simulink model "Sim_PD_XY"  (R2016a)
settings: Solver=VariableStepAuto  StartTime=0.0  StopTime=10.0  RelTol=1e-3
undefined symbols (not defined in the file or in its folder): k_reg, k_s, T_n, T_r
settings Model: Creator=Florian  LastModifiedBy=Florian

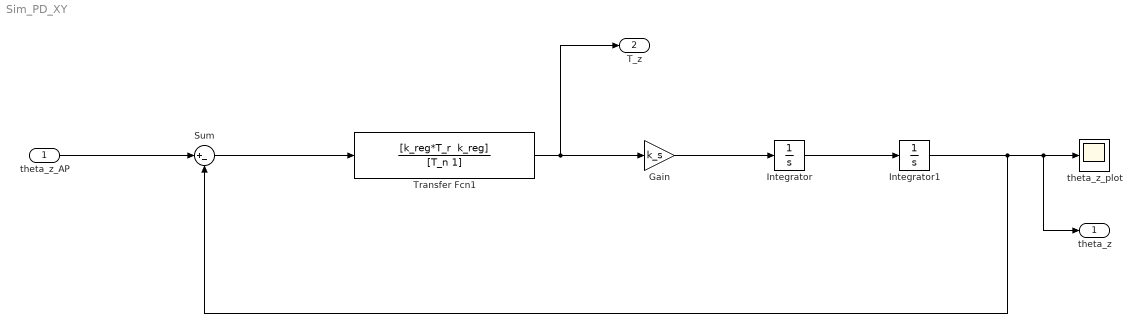
== system Sim_PD_XY ==
  "theta_z_AP " : Inport
  Gain : Gain  Gain=k_s
  Integrator : Integrator
  Integrator1 : Integrator  InitialCondition=pi/32
  Sum : Sum  Inputs=|+-
  Transfer Fcn1 : TransferFcn  Numerator="[k_reg*T_r  k_reg]"  Denominator=[T_n 1]
  theta_z_plot : Scope
  "theta_z " : Outport
  T_z : Outport  Port=2
  wires:
  Sum/1 -> Transfer Fcn1/1
  Transfer Fcn1/1 -> T_z/1, Gain/1
  Gain/1 -> Integrator/1
  Integrator/1 -> Integrator1/1
  Integrator1/1 -> "theta_z "/1, theta_z_plot/1, Sum/2
  "theta_z_AP "/1 -> Sum/1
